simulink model "Pendulum_Oscillator"  (R2019a)
settings: Solver=VariableStepAuto  StartTime=0.0  StopTime=10  MaxStep=0.01  RelTol=1e-3
model workspace (MAT data in the model file):
  I0 = 0.088
  L = 0.43
  g = 9.81
  m = 1
settings Model: Creator=91839  LastModifiedBy=91839
settings DataIOCC: ExternalInput=data  LoadExternalInput=on  SaveFormat=Array  DSMLogging=off  ReturnWorkspaceOutputs=off
settings DebuggingCC: SFMachineParentedDataDiag=error

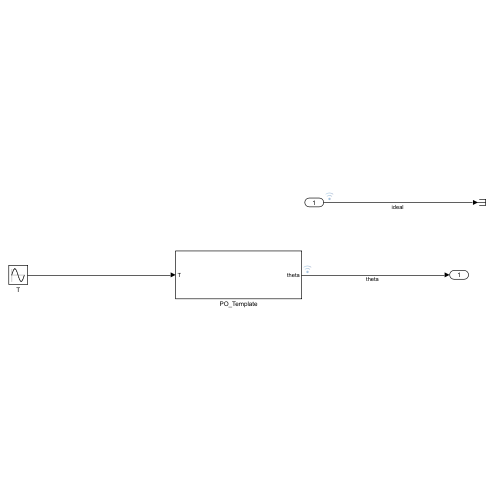
[thumbnail: Simulink's stored preview of the top-level diagram]
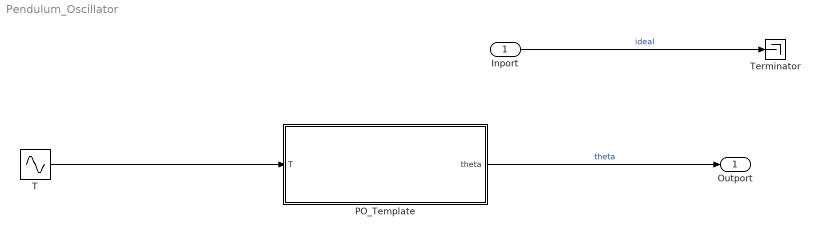
== system Pendulum_Oscillator ==
  Inport : Inport
  PO_Template : Subsystem
  T : Sin  SampleTime=0
  Terminator : Terminator
  Outport : Outport
  wires:
  Inport/1 -> Terminator/1  "ideal"
  T/1 -> PO_Template/1(T)
  PO_Template/1(theta) -> Outport/1  "theta"

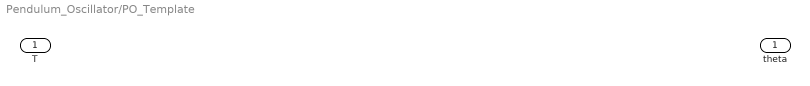
== system Pendulum_Oscillator/PO_Template ==
  T : Inport
  theta : Outport
